simulink model "step3"  (R2018b)
settings: Solver=VariableStepAuto  StartTime=0.0  StopTime=1000  RelTol=1e-3
values from neighbouring files (symbols this model uses):
  Ts = K(i)    [step3part2.m]    (also in step4part1.m = 10; step4part2.m = 10; step5part2.m = 10; step5part3.m = 10)
libraries: powerlib_meascontrol x1
settings Model: Creator=Asus  LastModifiedBy=Asus

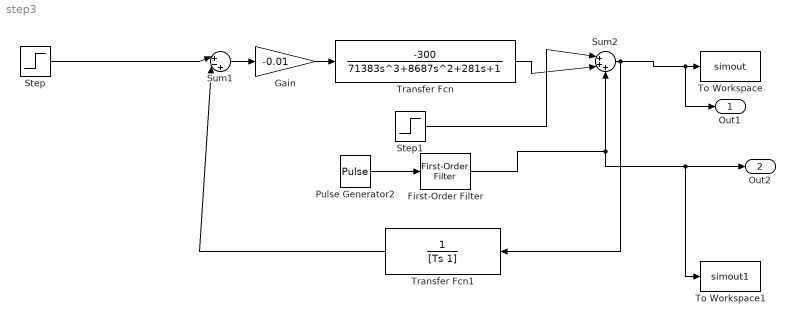
== system step3 ==
  First-Order Filter : powerlib_meascontrol/Filters/First-Order Filter  FilterType=Lowpass  Tc=50  Ts=0  Initialize=on  Vac_Init=[0, 0, 2]  Vdc_Init=0  PlotResponse=off  FreqRange="[0,  200,  1]"
      settings: SourceProductName=Simscape Power Systems
  Gain : Gain  Gain=-0.01
  Pulse Generator2 : DiscretePulseGenerator  PulseType=Time based  Amplitude=90  Period=1000  PulseWidth=10  PhaseDelay=30
  Step : Step  After=110  SampleTime=0
  Step1 : Step  After=110  SampleTime=0
  Sum1 : Sum  Inputs=|+-+
  Sum2 : Sum  Inputs=|+++
  To Workspace : ToWorkspace  VariableName=simout  SaveFormat=Timeseries  SampleTime=-1
  To Workspace1 : ToWorkspace  VariableName=simout1  SaveFormat=Timeseries  SampleTime=-1
  Transfer Fcn : TransferFcn  Numerator=[-300]  Denominator=[71383 8687 281 1]
  Transfer Fcn1 : TransferFcn  Denominator=[Ts 1]
  Out1 : Outport
  Out2 : Outport  Port=2
  wires:
  Transfer Fcn1/1 -> Sum1/2
  Sum1/1 -> Gain/1
  Gain/1 -> Transfer Fcn/1
  Step/1 -> Sum1/1
  Pulse Generator2/1 -> First-Order Filter/1
  Step1/1 -> Sum2/1
  Transfer Fcn/1 -> Sum2/2
  Sum2/1 -> Transfer Fcn1/1, Out1/1, To Workspace/1
  First-Order Filter/1 -> To Workspace1/1, Out2/1, Sum2/3
